simulink model "drone_simulation_3D"  (R2022b)
settings: Solver=VariableStepAuto  StartTime=0.0  StopTime=51  FixedStep=0.01  MaxStep=0.001  MinStep=0.00001  RelTol=1e-3
libraries: slpidlib x2, robotcorelib x1
settings Model: Creator=andre  LastModifiedBy=andre

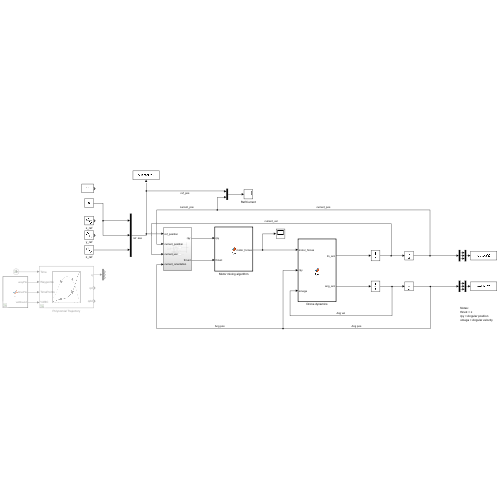
[thumbnail: Simulink's stored preview of the top-level diagram]
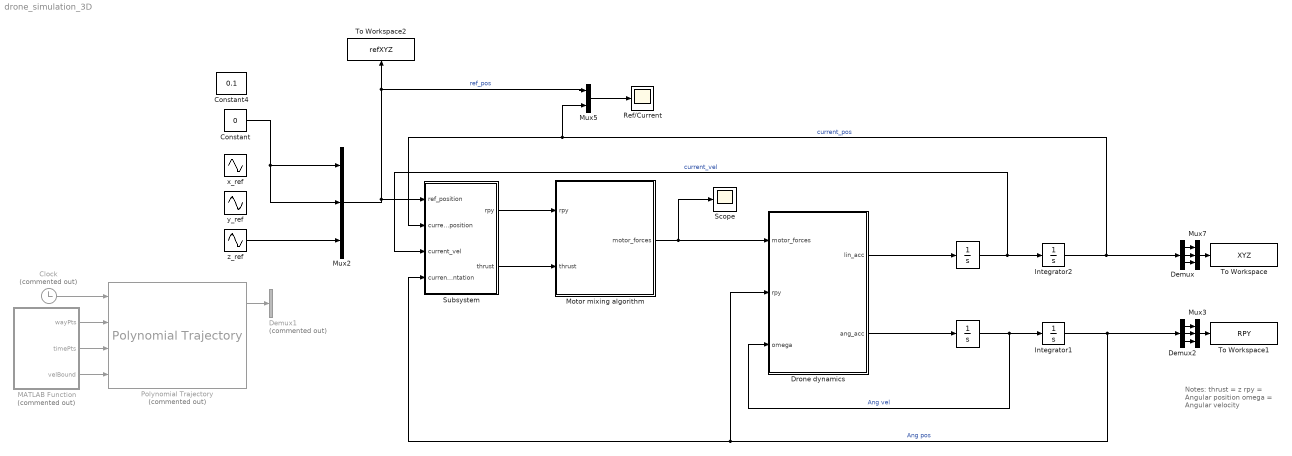
== system drone_simulation_3D ==
  note: Notes:
      | thrust = z
      | rpy = Angular position
      | omega = Angular velocity
  " " : Integrator  InitialCondition=[0 0 0]
  "  " : Integrator  InitialCondition=[0 0 0]
  Clock : Clock  Commented=on
  Constant : Constant  Value=0
  Constant4 : Constant  Value=0.1
  Demux : Demux  Outputs=3
  Demux1 : Demux  Commented=on  Outputs=3
  Demux2 : Demux  Outputs=3
  Drone dynamics : MATLAB Function  TreatAsAtomicUnit=on
  Integrator1 : Integrator
  Integrator2 : Integrator
  MATLAB Function : MATLAB Function  Commented=on  TreatAsAtomicUnit=on
  Motor mixing algorithm : MATLAB Function  TreatAsAtomicUnit=on
  Mux2 : Mux  Inputs=3
  Mux3 : Mux  Inputs=3
  Mux5 : Mux  Inputs=2
  Mux7 : Mux  Inputs=3
  Polynomial Trajectory : robotcorelib/Polynomial Trajectory  Commented=on  WaypointSource=External  Waypoints=[ 0, 2, 1, 5, 0]  TimePoints=[ 0, 1, 2, 3, 4 ]  TimeInterval=[ 1, 4 ]  Method=Cubic Polynomial  ParameterSource=External  VelocityBoundaryCondition=zeros( 1, 5 )  AccelerationBoundaryCondition=zeros( 2, 5 )  SimulateUsing=Interpreted execution
  Ref/Current : Scope
  Scope : Scope
  Subsystem : Subsystem
  To Workspace : ToWorkspace  VariableName=XYZ  SampleTime=-1
  To Workspace1 : ToWorkspace  VariableName=RPY  SampleTime=-1
  To Workspace2 : ToWorkspace  VariableName=refXYZ  SampleTime=-1
  x_ref : Sin  Amplitude=0.5  Frequency=0.5  SampleTime=0
  y_ref : Sin  Amplitude=0.4  Frequency=0.3  SampleTime=0
  z_ref : Sin  Amplitude=1.4  Frequency=0.5  SampleTime=0
  wires:
  Drone dynamics/1(lin_acc) -> " "/1
  Drone dynamics/2(ang_acc) -> "  "/1
  "  "/1 -> Drone dynamics/3(omega), Integrator1/1  "Ang vel"
  Integrator1/1 -> Drone dynamics/2(rpy), Subsystem/4(current_orientation), Demux2/1  "Ang pos"
  " "/1 -> Subsystem/3(current_vel), Integrator2/1  "current_vel"
  Integrator2/1 -> Mux5/2, Subsystem/2(current_position), Demux/1  "current_pos"
  Subsystem/1(rpy) -> Motor mixing algorithm/1(rpy)
  Subsystem/2(thrust) -> Motor mixing algorithm/2(thrust)
  Motor mixing algorithm/1(motor_forces) -> Scope/1, Drone dynamics/1(motor_forces)
  Mux5/1 -> Ref/Current/1
  Demux/1 -> Mux7/1
  Demux/2 -> Mux7/2
  Demux/3 -> Mux7/3
  Mux7/1 -> To Workspace/1
  MATLAB Function/2(timePts) -> Polynomial Trajectory/3
  MATLAB Function/3(velBound) -> Polynomial Trajectory/4
  MATLAB Function/1(wayPts) -> Polynomial Trajectory/2
  Clock/1 -> Polynomial Trajectory/1
  Mux2/1 -> Mux5/1, To Workspace2/1, Subsystem/1(ref_position)  "ref_pos"
  Polynomial Trajectory/1 -> Demux1/1
  Constant/1 -> Mux2/1, Mux2/2
  Demux2/3 -> Mux3/3
  Demux2/2 -> Mux3/2
  Demux2/1 -> Mux3/1
  Mux3/1 -> To Workspace1/1
  z_ref/1 -> Mux2/3

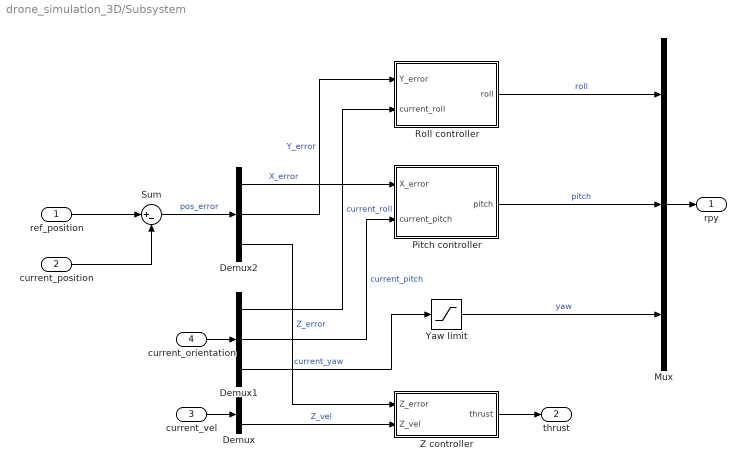
== system drone_simulation_3D/Subsystem ==
  ref_position : Inport
  current_position : Inport  Port=2
  current_vel : Inport  Port=3
  current_orientation : Inport  Port=4
  Demux : Demux  Outputs=3
  Demux1 : Demux  Outputs=3
  Demux2 : Demux  Outputs=3
  Mux : Mux  Inputs=3
  Pitch controller : Subsystem
  Roll controller : Subsystem
  Sum : Sum  Inputs=|+-
  Yaw limit : Saturate  UpperLimit=0  LowerLimit=0
  Z controller : Subsystem
  rpy : Outport
  thrust : Outport  Port=2
  wires:
  current_orientation/1 -> Demux1/1
  Mux/1 -> rpy/1
  Pitch controller/1(pitch) -> Mux/2  "pitch"
  Roll controller/1(roll) -> Mux/1  "roll"
  ref_position/1 -> Sum/1
  current_position/1 -> Sum/2
  Sum/1 -> Demux2/1  "pos_error"
  Demux2/1 -> Pitch controller/1(X_error)  "X_error"
  Demux2/2 -> Roll controller/1(Y_error)  "Y_error"
  Demux2/3 -> Z controller/1(Z_error)  "Z_error"
  Demux1/1 -> Roll controller/2(current_roll)  "current_roll"
  Demux1/2 -> Pitch controller/2(current_pitch)  "current_pitch"
  Yaw limit/1 -> Mux/3  "yaw"
  Demux1/3 -> Yaw limit/1  "current_yaw"
  current_vel/1 -> Demux/1
  Demux/3 -> Z controller/2(Z_vel)  "Z_vel"
  Z controller/1(thrust) -> thrust/1

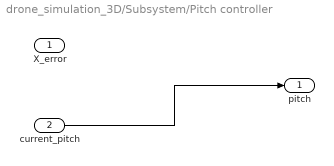
== system drone_simulation_3D/Subsystem/Pitch controller ==
  X_error : Inport
  current_pitch : Inport  Port=2
  pitch : Outport
  wires:
  current_pitch/1 -> pitch/1

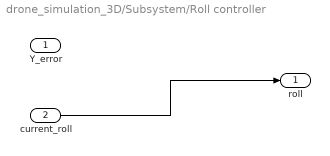
== system drone_simulation_3D/Subsystem/Roll controller ==
  Y_error : Inport
  current_roll : Inport  Port=2
  roll : Outport
  wires:
  current_roll/1 -> roll/1

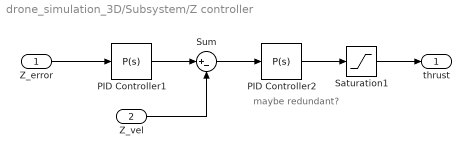
== system drone_simulation_3D/Subsystem/Z controller ==
  note: maybe redundant?
  Z_error : Inport
  Z_vel : Inport  Port=2
  PID Controller1 : slpidlib/PID Controller  Controller=P  Form=Parallel  TimeDomain=Continuous-time  UseExternalTs=off  SampleTime=-1  IntegratorMethod=Forward Euler  FilterMethod=Forward Euler  ControllerParametersSource=internal  P=17  I=1  UseKiTs=off  D=0  N=100  UseFilter=on  TunerSelectOption=Transfer Function Based (PID Tuner App)  InitialConditionSource=internal  InitialConditionForIntegrator=0  InitialConditionForFilter=0  DifferentiatorICPrevScaledInput=0  ExternalReset=none  TrackingMode=off  Kt=1  LimitOutput=off  SatLimitsSource=internal  UpperSaturationLimit=inf  LowerSaturationLimit=-inf  LinearizeAsGain=on  AntiWindupMode=none  Kb=1  LimitIntegrator=off  UpperIntegratorSaturationLimit=inf  LowerIntegratorSaturationLimit=-inf  POutMin=[]  POutMax=[]  IOutMin=[]  IOutMax=[]  DOutMin=[]  DOutMax=[]  NOutMin=[]  NOutMax=[]  SumOutMin=[]  SumOutMax=[]  SaturationOutMin=[]  SaturationOutMax=[]  PParamMin=[]  PParamMax=[]  IParamMin=[]  IParamMax=[]  DParamMin=[]  DParamMax=[]  NParamMin=[]  NParamMax=[]  KbParamMin=[]  KbParamMax=[]  KtParamMin=[]  KtParamMax=[]  KbOutMin=[]  KbOutMax=[]  KtOutMin=[]  KtOutMax=[]  IntegratorOutMin=[]  IntegratorOutMax=[]  FilterOutMin=[]  FilterOutMax=[]  SumI1OutMin=[]  SumI1OutMax=[]  SumI2OutMin=[]  SumI2OutMax=[]  SumI3OutMin=[]  SumI3OutMax=[]  SumI4OutMin=[]  SumI4OutMax=[]  SumDOutMin=[]  SumDOutMax=[]  DifferentiatorOutMin=[]  DifferentiatorOutMax=[]  FilterDiffOutCoefMin=[]  FilterDiffOutCoefMax=[]  ReciprocalOutMin=[]  ReciprocalOutMax=[]  SumDenOutMin=[]  SumDenOutMax=[]  SumNumOutMin=[]  SumNumOutMax=[]  DivideOutMin=[]  DivideOutMax=[]  UdiffTsProdOutMin=[]  UdiffTsProdOutMax=[]  NTsProdOutMin=[]  NTsProdOutMax=[]  UintegralTsProdOutMin=[]  UintegralTsProdOutMax=[]  UngainTsProdOutMin=[]  UngainTsProdOutMax=[]  ClampingZeroOutDataTypeStr=Inherit: Inherit via back propagation  ClampingZeroOutMin=[]  ClampingZeroOutMax=[]  FilterDenConstantOutDataTypeStr=Inherit: Inherit via back propagation  FilterDenConstantOutMin=[]  FilterDenConstantOutMax=[]  PCopyOutDataTypeStr=Inherit: Inherit via back propagation  PCopyOutMin=[]  PCopyOutMax=[]  NCopyOutDataTypeStr=Inherit: Inherit via back propagation  NCopyOutMin=[]  NCopyOutMax=[]  IntegratorContinuousStateAttributes=''  IntegratorStateMustResolveToSignalObject=off  IntegratorRTWStateStorageClass=Auto  FilterContinuousStateAttributes=''  FilterStateMustResolveToSignalObject=off  FilterRTWStateStorageClass=Auto  ParallelPVariant=InternalParameters  IdealPVariant=Disabled  IVariant=Disabled  DVariant=Disabled  IntegratorVariant=Disabled  SatVariant=Disabled  AWVariant=Disabled  PCopyVariant=Disabled  TRVariant=Disabled  FdbkBlocksVariant=Forward  IdealPFdbkVariant=Disabled  SatFdbkVariant=Disabled  DerivativeFilterVariant=Disabled  NVariant=Disabled  NCopyVariant=Disabled_SignalSpec  FilterICVariant=Disabled  IntegratorICVariant=Disabled  ExternalResetVariant=Disabled  TRSumVariant=Passthrough  SumFdbkVariant=Disabled  SumVariant=Passthrough_P  TsampFilterVariant=InternalTs  TsampNgainVariant=Passthrough  TsampIntegralVariant=Disabled_SignalSpec  ExternalSaturationOutDataTypeStr=Inherit: Same as second input
  PID Controller2 : slpidlib/PID Controller  Controller=P  Form=Parallel  TimeDomain=Continuous-time  UseExternalTs=off  SampleTime=-1  IntegratorMethod=Forward Euler  FilterMethod=Forward Euler  ControllerParametersSource=internal  P=0.8  I=1  UseKiTs=off  D=0  N=100  UseFilter=on  TunerSelectOption=Transfer Function Based (PID Tuner App)  InitialConditionSource=internal  InitialConditionForIntegrator=0  InitialConditionForFilter=0  DifferentiatorICPrevScaledInput=0  ExternalReset=none  TrackingMode=off  Kt=1  LimitOutput=off  SatLimitsSource=internal  UpperSaturationLimit=inf  LowerSaturationLimit=-inf  LinearizeAsGain=on  AntiWindupMode=none  Kb=1  LimitIntegrator=off  UpperIntegratorSaturationLimit=inf  LowerIntegratorSaturationLimit=-inf  POutMin=[]  POutMax=[]  IOutMin=[]  IOutMax=[]  DOutMin=[]  DOutMax=[]  NOutMin=[]  NOutMax=[]  SumOutMin=[]  SumOutMax=[]  SaturationOutMin=[]  SaturationOutMax=[]  PParamMin=[]  PParamMax=[]  IParamMin=[]  IParamMax=[]  DParamMin=[]  DParamMax=[]  NParamMin=[]  NParamMax=[]  KbParamMin=[]  KbParamMax=[]  KtParamMin=[]  KtParamMax=[]  KbOutMin=[]  KbOutMax=[]  KtOutMin=[]  KtOutMax=[]  IntegratorOutMin=[]  IntegratorOutMax=[]  FilterOutMin=[]  FilterOutMax=[]  SumI1OutMin=[]  SumI1OutMax=[]  SumI2OutMin=[]  SumI2OutMax=[]  SumI3OutMin=[]  SumI3OutMax=[]  SumI4OutMin=[]  SumI4OutMax=[]  SumDOutMin=[]  SumDOutMax=[]  DifferentiatorOutMin=[]  DifferentiatorOutMax=[]  FilterDiffOutCoefMin=[]  FilterDiffOutCoefMax=[]  ReciprocalOutMin=[]  ReciprocalOutMax=[]  SumDenOutMin=[]  SumDenOutMax=[]  SumNumOutMin=[]  SumNumOutMax=[]  DivideOutMin=[]  DivideOutMax=[]  UdiffTsProdOutMin=[]  UdiffTsProdOutMax=[]  NTsProdOutMin=[]  NTsProdOutMax=[]  UintegralTsProdOutMin=[]  UintegralTsProdOutMax=[]  UngainTsProdOutMin=[]  UngainTsProdOutMax=[]  ClampingZeroOutDataTypeStr=Inherit: Inherit via back propagation  ClampingZeroOutMin=[]  ClampingZeroOutMax=[]  FilterDenConstantOutDataTypeStr=Inherit: Inherit via back propagation  FilterDenConstantOutMin=[]  FilterDenConstantOutMax=[]  PCopyOutDataTypeStr=Inherit: Inherit via back propagation  PCopyOutMin=[]  PCopyOutMax=[]  NCopyOutDataTypeStr=Inherit: Inherit via back propagation  NCopyOutMin=[]  NCopyOutMax=[]  IntegratorContinuousStateAttributes=''  IntegratorStateMustResolveToSignalObject=off  IntegratorRTWStateStorageClass=Auto  FilterContinuousStateAttributes=''  FilterStateMustResolveToSignalObject=off  FilterRTWStateStorageClass=Auto  ParallelPVariant=InternalParameters  IdealPVariant=Disabled  IVariant=Disabled  DVariant=Disabled  IntegratorVariant=Disabled  SatVariant=Disabled  AWVariant=Disabled  PCopyVariant=Disabled  TRVariant=Disabled  FdbkBlocksVariant=Forward  IdealPFdbkVariant=Disabled  SatFdbkVariant=Disabled  DerivativeFilterVariant=Disabled  NVariant=Disabled  NCopyVariant=Disabled_SignalSpec  FilterICVariant=Disabled  IntegratorICVariant=Disabled  ExternalResetVariant=Disabled  TRSumVariant=Passthrough  SumFdbkVariant=Disabled  SumVariant=Passthrough_P  TsampFilterVariant=InternalTs  TsampNgainVariant=Passthrough  TsampIntegralVariant=Disabled_SignalSpec  ExternalSaturationOutDataTypeStr=Inherit: Same as second input
  Saturation1 : Saturate  UpperLimit=(57.9/1000) * 9.82  LowerLimit=0
  Sum : Sum  Inputs=|+-
  thrust : Outport
  wires:
  Z_error/1 -> PID Controller1/1
  Sum/1 -> PID Controller2/1
  PID Controller1/1 -> Sum/1
  Saturation1/1 -> thrust/1
  Z_vel/1 -> Sum/2
  PID Controller2/1 -> Saturation1/1

== matlab function drone_simulation_3D/Motor mixing algorithm ==
  data: motor_forces output size=[1, 4]; rpy input size=[1, 3]; thrust input
function motor_forces = fcn(rpy, thrust)

% r = rpy(1);
% p = rpy(2);
% y = rpy(3);
% z = thrust;
% 
% motor_forces = ...
% [sum([r -p y z]); ...
% sum([-r -p -y z]);   ...
% sum([-r p y z]);   ...
% sum([r p -y z])];

m1 = thrust + rpy(1) + rpy(2) + rpy(3);
m2 = thrust - rpy(1) + rpy(2) - rpy(3);
m3 = thrust - rpy(1) - rpy(2) - rpy(3);
m4 = thrust + rpy(1) - rpy(2) + rpy(3);
motor_forces = [m1, m2, m3, m4];

== matlab function drone_simulation_3D/Drone dynamics ==
  data: motor_forces input; lin_acc output; rpy input; ang_acc output; omega input
function [lin_acc, ang_acc] = fcn(motor_forces, rpy, omega)

%% Define constants
rotor_dist = 0.04; %m
body_mass = 0.02989; %kg
g_constant = [0;0;-9.82]; %Nm/s^2

% Vectors from CoM to motors
% We create a X-configured drone
rotor_angle = pi/4;
s1 = [cos(rotor_angle); sin(rotor_angle); 0] * rotor_dist;
s2 = [cos(rotor_angle); -sin(rotor_angle); 0] * rotor_dist;
s3 = [-cos(rotor_angle); -sin(rotor_angle); 0] * rotor_dist;
s4 = [-cos(rotor_angle); sin(rotor_angle); 0] * rotor_dist;
s_vectors = [s1 s2 s3 s4];

% Local motor force vectors
m1_vec = [0;0;motor_forces(1)];
m2_vec = [0;0;motor_forces(2)];
m3_vec = [0;0;motor_forces(3)];
m4_vec = [0;0;motor_forces(4)];
local_motor_forces = [m1_vec m2_vec m3_vec m4_vec];

% Local inertia tensor
I_local = [1.132869584e-05 0 0; 0 1.132869584e-05 0; 0 0 2.028869584e-05];



%% Calculate drone components

% Rotation matrix
%R = rpy2r(rpy(1), rpy(2), rpy(3));
R = rotx(rpy(1)) * roty(rpy(2)) * rotz(rpy(3));

% Global inertia tensor
I_global = (R * I_local) * transpose(R);


%% Equation of motion

% Total force
total_force = R * sum(local_motor_forces,2) + (body_mass * g_constant);

% Total moment
total_moment = R * sum(cross(s_vectors,local_motor_forces),2);

%% Linear and angular acceleration
a = total_force/body_mass;
lin_acc = [a(1) a(2) a(3)];

alpha = inv(I_global) * (total_moment - cross(omega,(I_global * omega)));
ang_acc = [alpha(1) alpha(2) alpha(3)];
% omega = angular velocity
% alpha = angular acceleration

== matlab function drone_simulation_3D/MATLAB Function ==
  data: wayPts output; timePts output; velBound output
function [wayPts,timePts,velBound] = fcn()

xPts = [0,1,1,-1,-1,0];
yPts = [0,1,-1,-1,1,0];
zPts = [0,1,2,3,4,5];

wayPts = [xPts;yPts;zPts];
timePts = [0,10,20,30,40,50];


%velBound = ones(size(wayPts)) * 0.1;
velBound = zeros(size(wayPts));
